simulink model "topic_sub"  (R2020b)
settings: Solver=FixedStepAuto  StartTime=0.0  StopTime=inf  RelTol=1e-3
undefined symbols (not defined in the file): BodyRate, Header, Orientation, Pose, Twist
libraries: robotlib x33, pid_lib x4
settings Model: Creator=mario  LastModifiedBy=mario
settings OptimizationCC: DefaultParameterBehavior=Inlined  EnhancedBackFolding=on  PassReuseOutputArgsAs=Individual arguments  ZeroExternalMemoryAtStartup=off  ZeroInternalMemoryAtStartup=off  InitFltsAndDblsToZero=on  MaxStackSize=64  OptimizeBlockOrder=speed  DifferentSizesBufferReuse=on  OptimizationCustomize=off  EfficientTunableParamExpr=on
settings DebuggingCC: ParameterTunabilityLossMsg=error
settings HardwareCC: ProdBitPerPointer=32  ProdBitPerSizeT=32  ProdBitPerPtrDiffT=32  ProdLargestAtomicFloat=None  ProdIntDivRoundTo=Undefined  ProdEndianess=Unspecified  ProdWordSize=32  ProdLongLongMode=on  ProdHWDeviceType=Generic->Unspecified (assume 32-bit Generic)  TargetLongLongMode=on
settings SFSimCC: MATLABDynamicMemAlloc=off
settings RTWCC: Description=Embedded Coder  SystemTargetFile=ert.tlc  HardwareBoard=Robot Operating System (ROS)  TLCOptions="-aInlineSetEventsForThisBaseRateFcn=TLC_FALSE -aSuppressMultiTaskScheduler=TLC_FALSE  -aRateBasedStepFcn=0"  GenCodeOnly=on  TemplateMakefile=ert_default_tmf  Toolchain=Catkin  TargetLang=C++  GenerateGPUCode=CUDA
settings CodeAppCC: ForceParamTrailComments=on  IgnoreCustomStorageClasses=off  OperatorAnnotations=on  SimulinkDataObjDesc=on  SFDataObjDesc=on  InsertBlockDesc=on
settings ERTTargetCC: CodeInterfacePackaging=C++ class  InlinedParameterPlacement=NonHierarchical  RootIOFormat=Structure reference  ERTCustomFileTemplate=example_file_process.tlc

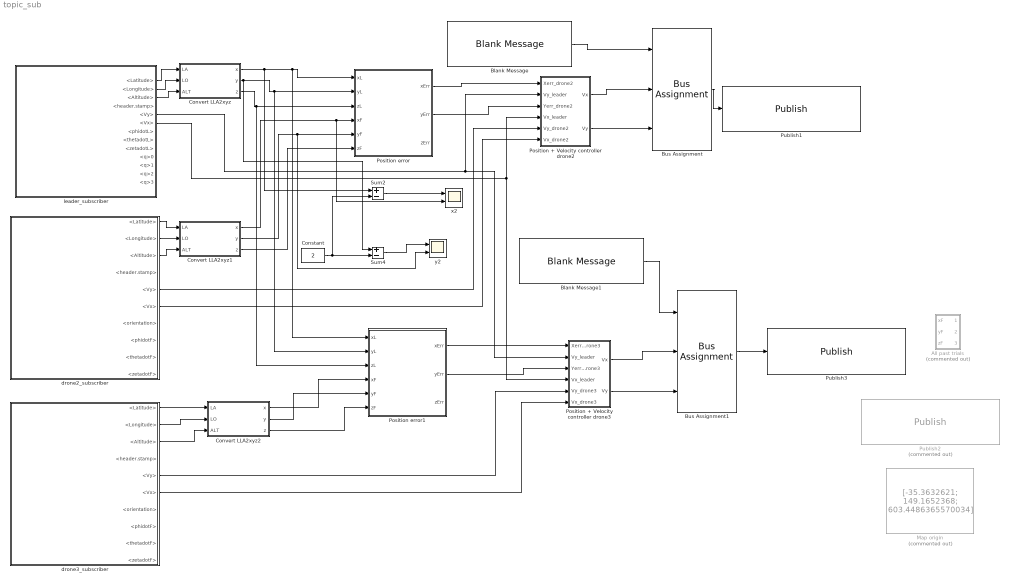
== system topic_sub ==
  All past trials : Subsystem  Commented=on
  Blank Message : robotlib/Blank Message  messageClass=Message  entityType=geometry_msgs/TwistStamped  messageType=geometry_msgs/TwistStamped  SampleTime=inf  legacyBusStruct=off
  Blank Message1 : robotlib/Blank Message  messageClass=Message  entityType=geometry_msgs/TwistStamped  messageType=geometry_msgs/TwistStamped  SampleTime=inf  legacyBusStruct=off
  Bus Assignment : BusAssignment  AssignedSignals=Twist.Linear.X,Twist.Linear.Y
  Bus Assignment1 : BusAssignment  AssignedSignals=Twist.Linear.X,Twist.Linear.Y
  Constant : Constant  Value=2
  Convert LLA2xyz : MATLAB Function  TreatAsAtomicUnit=on
  Convert LLA2xyz1 : MATLAB Function  TreatAsAtomicUnit=on
  Convert LLA2xyz2 : MATLAB Function  TreatAsAtomicUnit=on
  Map origin : Constant  Commented=on  Value=[-35.3632621; 149.1652368; 603.4486365570034]  VectorParams1D=off  SampleTime=-1
  Position + Velocity controller drone2 : Subsystem
  Position + Velocity controller drone3 : Subsystem
  Position error : MATLAB Function  TreatAsAtomicUnit=on
  Position error1 : MATLAB Function  TreatAsAtomicUnit=on
  Publish1 : robotlib/Publish  topicSource=Select from ROS network  topic=/drone2/mavros/setpoint_velocity/cmd_vel  messageType=geometry_msgs/TwistStamped  legacyBusStruct=off  messageQueueLength=1
  Publish2 : robotlib/Publish  Commented=on  topicSource=Select from ROS network  topic=/drone2/mavros/setpoint_velocity/cmd_vel  messageType=geometry_msgs/TwistStamped  legacyBusStruct=off  messageQueueLength=1
  Publish3 : robotlib/Publish  topicSource=Select from ROS network  topic=/drone3/mavros/setpoint_velocity/cmd_vel  messageType=geometry_msgs/TwistStamped  legacyBusStruct=off  messageQueueLength=1
  Sum2 : Sum  Inputs=+-
  Sum4 : Sum  Inputs=+-
  drone2_subscriber : Subsystem
  drone3_subscriber : Subsystem
  leader_subscriber : Subsystem
  x2 : Scope  NumInputPorts=2
  y2 : Scope  NumInputPorts=2
  wires:
  Blank Message/1 -> Bus Assignment/1
  Bus Assignment/1 -> Publish1/1
  leader_subscriber/1(<Latitude>) -> Convert LLA2xyz/1(LA)
  leader_subscriber/2(<Longitude>) -> Convert LLA2xyz/2(LO)
  leader_subscriber/3(<Altitude>) -> Convert LLA2xyz/3(ALT)
  Convert LLA2xyz/1(x) -> Sum2/1, Position error1/1(xL), Position error/1(xL)
  Convert LLA2xyz/2(y) -> Sum4/1, Position error1/2(yL), Position error/2(yL)
  Convert LLA2xyz/3(z) -> Position error1/3(zL), Position error/3(zL)
  drone2_subscriber/2(<Longitude>) -> Convert LLA2xyz1/2(LO)
  drone2_subscriber/1(<Latitude>) -> Convert LLA2xyz1/1(LA)
  drone2_subscriber/3(<Altitude>) -> Convert LLA2xyz1/3(ALT)
  Convert LLA2xyz1/1(x) -> x2/2, Position error/4(xF)
  Convert LLA2xyz1/2(y) -> Position error/5(yF), y2/2
  Convert LLA2xyz1/3(z) -> Position error/6(zF)
  Constant/1 -> Sum2/2, Sum4/2
  Position error/1(xErr) -> Position + Velocity controller drone2/1(Xerr_drone2)
  leader_subscriber/5(<Vy>) -> Position + Velocity controller drone2/2(Vy_leader), Position + Velocity controller drone3/2(Vy_leader)
  Position error/2(yErr) -> Position + Velocity controller drone2/3(Yerr_drone2)
  leader_subscriber/6(<Vx>) -> Position + Velocity controller drone3/4(Vx_leader), Position + Velocity controller drone2/4(Vx_leader)
  drone2_subscriber/5(<Vy>) -> Position + Velocity controller drone2/5(Vy_drone2)
  drone2_subscriber/6(<Vx>) -> Position + Velocity controller drone2/6(Vx_drone2)
  Position + Velocity controller drone2/1(Vx) -> Bus Assignment/2
  Position + Velocity controller drone2/2(Vy) -> Bus Assignment/3
  Sum2/1 -> x2/1
  Sum4/1 -> y2/1
  drone3_subscriber/1(<Latitude>) -> Convert LLA2xyz2/1(LA)
  drone3_subscriber/2(<Longitude>) -> Convert LLA2xyz2/2(LO)
  drone3_subscriber/3(<Altitude>) -> Convert LLA2xyz2/3(ALT)
  Convert LLA2xyz2/1(x) -> Position error1/4(xF)
  Convert LLA2xyz2/2(y) -> Position error1/5(yF)
  Convert LLA2xyz2/3(z) -> Position error1/6(zF)
  Position error1/1(xErr) -> Position + Velocity controller drone3/1(Xerr_drone3)
  Position error1/2(yErr) -> Position + Velocity controller drone3/3(Yerr_drone3)
  Position + Velocity controller drone3/1(Vx) -> Bus Assignment1/2
  Position + Velocity controller drone3/2(Vy) -> Bus Assignment1/3
  Bus Assignment1/1 -> Publish3/1
  Blank Message1/1 -> Bus Assignment1/1
  drone3_subscriber/5(<Vy>) -> Position + Velocity controller drone3/5(Vy_drone3)
  drone3_subscriber/6(<Vx>) -> Position + Velocity controller drone3/6(Vx_drone3)

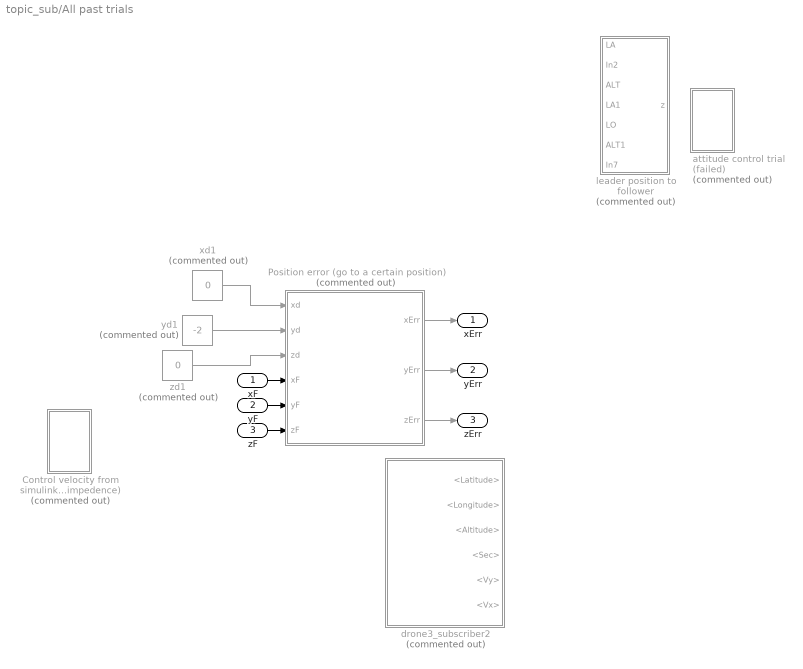
== system topic_sub/All past trials ==
  xF : Inport
  yF : Inport  Port=2
  zF : Inport  Port=3
  Control velocity from simulink trial(virtual impedence) : Subsystem  Commented=on
  Position error (go to a certain position) : MATLAB Function  Commented=on  TreatAsAtomicUnit=on
  attitude control trial (failed) : Subsystem  Commented=on
  drone3_subscriber2 : Subsystem  Commented=on
  leader position to follower : Subsystem  Commented=on
  xd1 : Constant  Commented=on  Value=0
  yd1 : Constant  Commented=on  Value=-2
  zd1 : Constant  Commented=on  Value=0
  xErr : Outport
  yErr : Outport  Port=2
  zErr : Outport  Port=3
  wires:
  Position error (go to a certain position)/3(zErr) -> zErr/1
  Position error (go to a certain position)/2(yErr) -> yErr/1
  xF/1 -> Position error (go to a certain position)/4(xF)
  zF/1 -> Position error (go to a certain position)/6(zF)
  yd1/1 -> Position error (go to a certain position)/2(yd)
  xd1/1 -> Position error (go to a certain position)/1(xd)
  Position error (go to a certain position)/1(xErr) -> xErr/1
  yF/1 -> Position error (go to a certain position)/5(yF)
  zd1/1 -> Position error (go to a certain position)/3(zd)

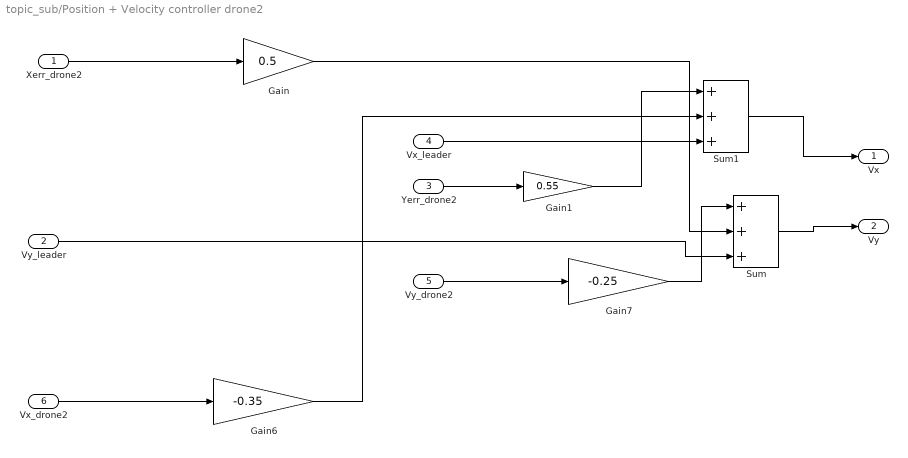
== system topic_sub/Position + Velocity controller drone2 ==
  Xerr_drone2 : Inport
  Vy_leader : Inport  Port=2
  Yerr_drone2 : Inport  Port=3
  Vx_leader : Inport  Port=4
  Vy_drone2 : Inport  Port=5
  Vx_drone2 : Inport  Port=6
  Gain : Gain  Gain=0.5
  Gain1 : Gain  Gain=0.55
  Gain6 : Gain  Gain=-0.35
  Gain7 : Gain  Gain=-0.25
  Sum : Sum  Inputs=+++
  Sum1 : Sum  Inputs=+++
  Vx : Outport
  Vy : Outport  Port=2
  wires:
  Vx_leader/1 -> Sum1/3
  Vy_leader/1 -> Sum/3
  Gain6/1 -> Sum1/2
  Vy_drone2/1 -> Gain7/1
  Gain7/1 -> Sum/1
  Sum/1 -> Vy/1
  Sum1/1 -> Vx/1
  Xerr_drone2/1 -> Gain/1
  Yerr_drone2/1 -> Gain1/1
  Gain1/1 -> Sum1/1
  Vx_drone2/1 -> Gain6/1
  Gain/1 -> Sum/2

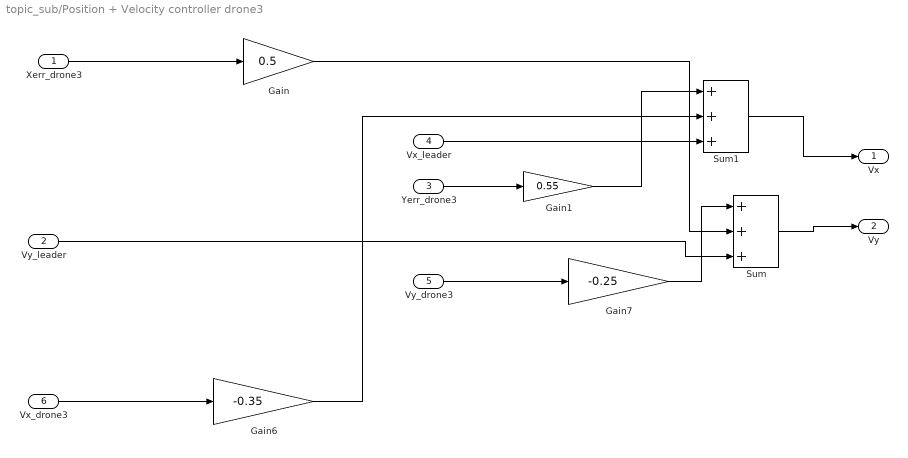
== system topic_sub/Position + Velocity controller drone3 ==
  Xerr_drone3 : Inport
  Vy_leader : Inport  Port=2
  Yerr_drone3 : Inport  Port=3
  Vx_leader : Inport  Port=4
  Vy_drone3 : Inport  Port=5
  Vx_drone3 : Inport  Port=6
  Gain : Gain  Gain=0.5
  Gain1 : Gain  Gain=0.55
  Gain6 : Gain  Gain=-0.35
  Gain7 : Gain  Gain=-0.25
  Sum : Sum  Inputs=+++
  Sum1 : Sum  Inputs=+++
  Vx : Outport
  Vy : Outport  Port=2
  wires:
  Gain/1 -> Sum/2
  Vx_drone3/1 -> Gain6/1
  Gain1/1 -> Sum1/1
  Yerr_drone3/1 -> Gain1/1
  Xerr_drone3/1 -> Gain/1
  Sum1/1 -> Vx/1
  Sum/1 -> Vy/1
  Gain7/1 -> Sum/1
  Vy_drone3/1 -> Gain7/1
  Gain6/1 -> Sum1/2
  Vy_leader/1 -> Sum/3
  Vx_leader/1 -> Sum1/3

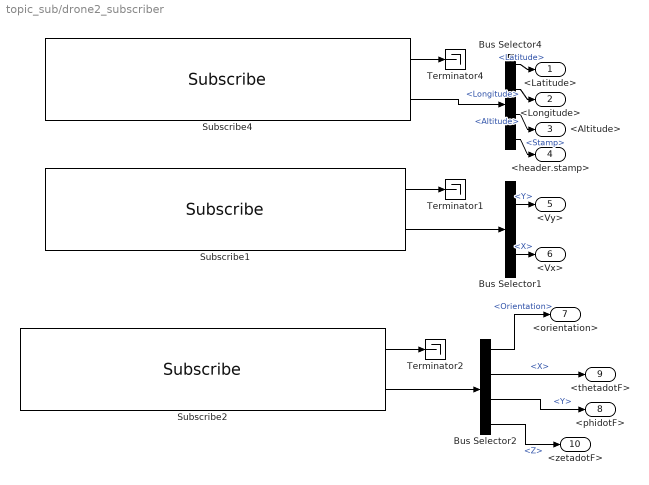
== system topic_sub/drone2_subscriber ==
  Bus Selector1 : BusSelector  OutputSignals=Twist.Linear.Y,Twist.Linear.X
  Bus Selector2 : BusSelector  OutputSignals=Orientation,AngularVelocity.X,AngularVelocity.Y,AngularVelocity.Z
  Bus Selector4 : BusSelector  OutputSignals=Latitude,Longitude,Altitude,Header.Stamp
  Subscribe1 : robotlib/Subscribe  topicSource=Select from ROS network  topic=/drone2/mavros/global_position/raw/gps_vel  messageType=geometry_msgs/TwistStamped  SampleTime=-1  legacyBusStruct=off  messageQueueLength=1
  Subscribe2 : robotlib/Subscribe  topicSource=Select from ROS network  topic=/drone2/mavros/imu/data  messageType=sensor_msgs/Imu  SampleTime=-1  legacyBusStruct=off  messageQueueLength=1
  Subscribe4 : robotlib/Subscribe  topicSource=Select from ROS network  topic=/drone2/mavros/global_position/raw/fix  messageType=sensor_msgs/NavSatFix  SampleTime=-1  legacyBusStruct=off  messageQueueLength=1
  Terminator1 : Terminator
  Terminator2 : Terminator
  Terminator4 : Terminator
  <Latitude> : Outport
  <Longitude> : Outport  Port=2
  <Altitude> : Outport  Port=3
  <header.stamp> : Outport  Port=4
  <Vy> : Outport  Port=5
  <Vx> : Outport  Port=6
  <orientation> : Outport  Port=7
  <phidotF> : Outport  Port=8
  <thetadotF> : Outport  Port=9
  <zetadotF> : Outport  Port=10
  wires:
  Bus Selector4/1 -> <Latitude>/1  "<Latitude>"
  Subscribe1/2 -> Bus Selector1/1
  Bus Selector1/2 -> <Vx>/1  "<X>"
  Subscribe4/1 -> Terminator4/1
  Bus Selector1/1 -> <Vy>/1  "<Y>"
  Bus Selector4/3 -> <Altitude>/1  "<Altitude>"
  Bus Selector4/2 -> <Longitude>/1  "<Longitude>"
  Subscribe1/1 -> Terminator1/1
  Subscribe4/2 -> Bus Selector4/1
  Bus Selector2/3 -> <phidotF>/1  "<Y>"
  Bus Selector2/4 -> <zetadotF>/1  "<Z>"
  Subscribe2/2 -> Bus Selector2/1
  Subscribe2/1 -> Terminator2/1
  Bus Selector2/2 -> <thetadotF>/1  "<X>"
  Bus Selector2/1 -> <orientation>/1  "<Orientation>"
  Bus Selector4/4 -> <header.stamp>/1  "<Stamp>"

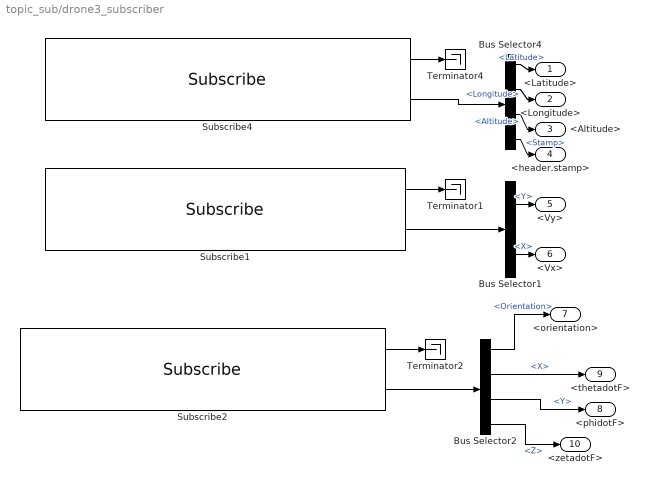
== system topic_sub/drone3_subscriber ==
  Bus Selector1 : BusSelector  OutputSignals=Twist.Linear.Y,Twist.Linear.X
  Bus Selector2 : BusSelector  OutputSignals=Orientation,AngularVelocity.X,AngularVelocity.Y,AngularVelocity.Z
  Bus Selector4 : BusSelector  OutputSignals=Latitude,Longitude,Altitude,Header.Stamp
  Subscribe1 : robotlib/Subscribe  topicSource=Select from ROS network  topic=/drone3/mavros/global_position/raw/gps_vel  messageType=geometry_msgs/TwistStamped  SampleTime=-1  legacyBusStruct=off  messageQueueLength=1
  Subscribe2 : robotlib/Subscribe  topicSource=Select from ROS network  topic=/drone3/mavros/imu/data  messageType=sensor_msgs/Imu  SampleTime=-1  legacyBusStruct=off  messageQueueLength=1
  Subscribe4 : robotlib/Subscribe  topicSource=Select from ROS network  topic=/drone3/mavros/global_position/raw/fix  messageType=sensor_msgs/NavSatFix  SampleTime=-1  legacyBusStruct=off  messageQueueLength=1
  Terminator1 : Terminator
  Terminator2 : Terminator
  Terminator4 : Terminator
  <Latitude> : Outport
  <Longitude> : Outport  Port=2
  <Altitude> : Outport  Port=3
  <header.stamp> : Outport  Port=4
  <Vy> : Outport  Port=5
  <Vx> : Outport  Port=6
  <orientation> : Outport  Port=7
  <phidotF> : Outport  Port=8
  <thetadotF> : Outport  Port=9
  <zetadotF> : Outport  Port=10
  wires:
  Bus Selector4/4 -> <header.stamp>/1  "<Stamp>"
  Bus Selector2/1 -> <orientation>/1  "<Orientation>"
  Bus Selector2/2 -> <thetadotF>/1  "<X>"
  Subscribe2/1 -> Terminator2/1
  Subscribe2/2 -> Bus Selector2/1
  Bus Selector2/4 -> <zetadotF>/1  "<Z>"
  Bus Selector2/3 -> <phidotF>/1  "<Y>"
  Subscribe4/2 -> Bus Selector4/1
  Subscribe1/1 -> Terminator1/1
  Bus Selector4/2 -> <Longitude>/1  "<Longitude>"
  Bus Selector4/3 -> <Altitude>/1  "<Altitude>"
  Bus Selector1/1 -> <Vy>/1  "<Y>"
  Subscribe4/1 -> Terminator4/1
  Bus Selector1/2 -> <Vx>/1  "<X>"
  Subscribe1/2 -> Bus Selector1/1
  Bus Selector4/1 -> <Latitude>/1  "<Latitude>"

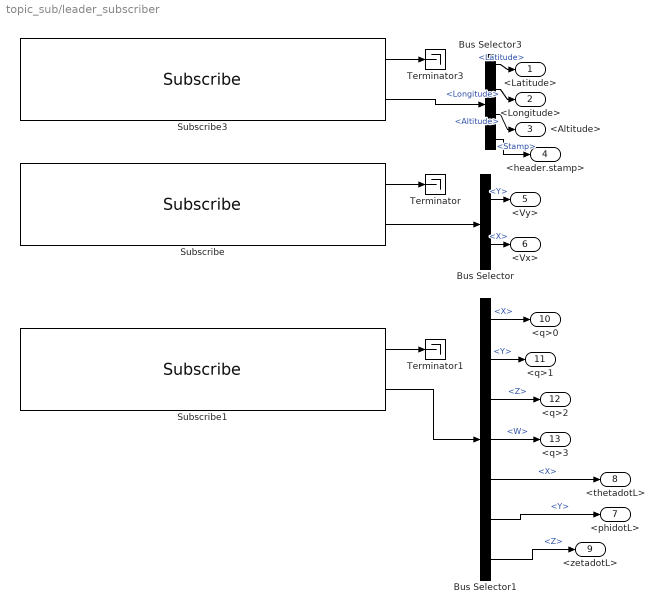
== system topic_sub/leader_subscriber ==
  Bus Selector : BusSelector  OutputSignals=Twist.Linear.Y,Twist.Linear.X
  Bus Selector1 : BusSelector  OutputSignals=Orientation.X,Orientation.Y,Orientation.Z,Orientation.W,AngularVelocity.X,AngularVelocity.Y,AngularVelocity.Z
  Bus Selector3 : BusSelector  OutputSignals=Latitude,Longitude,Altitude,Header.Stamp
  Subscribe : robotlib/Subscribe  topicSource=Select from ROS network  topic=/drone1/mavros/global_position/raw/gps_vel  messageType=geometry_msgs/TwistStamped  SampleTime=-1  legacyBusStruct=off  messageQueueLength=1
  Subscribe1 : robotlib/Subscribe  topicSource=Select from ROS network  topic=/drone1/mavros/imu/data  messageType=sensor_msgs/Imu  SampleTime=-1  legacyBusStruct=off  messageQueueLength=1
  Subscribe3 : robotlib/Subscribe  topicSource=Select from ROS network  topic=/drone1/mavros/global_position/raw/fix  messageType=sensor_msgs/NavSatFix  SampleTime=-1  legacyBusStruct=off  messageQueueLength=1000
  Terminator : Terminator
  Terminator1 : Terminator
  Terminator3 : Terminator
  <Latitude> : Outport
  <Longitude> : Outport  Port=2
  <Altitude> : Outport  Port=3
  <header.stamp> : Outport  Port=4
  <Vy> : Outport  Port=5
  <Vx> : Outport  Port=6
  <phidotL> : Outport  Port=7
  <thetadotL> : Outport  Port=8
  <zetadotL> : Outport  Port=9
  <q>0 : Outport  Port=10
  <q>1 : Outport  Port=11
  <q>2 : Outport  Port=12
  <q>3 : Outport  Port=13
  wires:
  Bus Selector3/3 -> <Altitude>/1  "<Altitude>"
  Subscribe3/1 -> Terminator3/1
  Subscribe3/2 -> Bus Selector3/1
  Bus Selector3/2 -> <Longitude>/1  "<Longitude>"
  Bus Selector/2 -> <Vx>/1  "<X>"
  Bus Selector3/1 -> <Latitude>/1  "<Latitude>"
  Subscribe/2 -> Bus Selector/1
  Bus Selector/1 -> <Vy>/1  "<Y>"
  Subscribe/1 -> Terminator/1
  Subscribe1/1 -> Terminator1/1
  Subscribe1/2 -> Bus Selector1/1
  Bus Selector1/5 -> <thetadotL>/1  "<X>"
  Bus Selector1/6 -> <phidotL>/1  "<Y>"
  Bus Selector1/7 -> <zetadotL>/1  "<Z>"
  Bus Selector1/1 -> <q>0/1  "<X>"
  Bus Selector1/2 -> <q>1/1  "<Y>"
  Bus Selector1/3 -> <q>2/1  "<Z>"
  Bus Selector1/4 -> <q>3/1  "<W>"
  Bus Selector3/4 -> <header.stamp>/1  "<Stamp>"

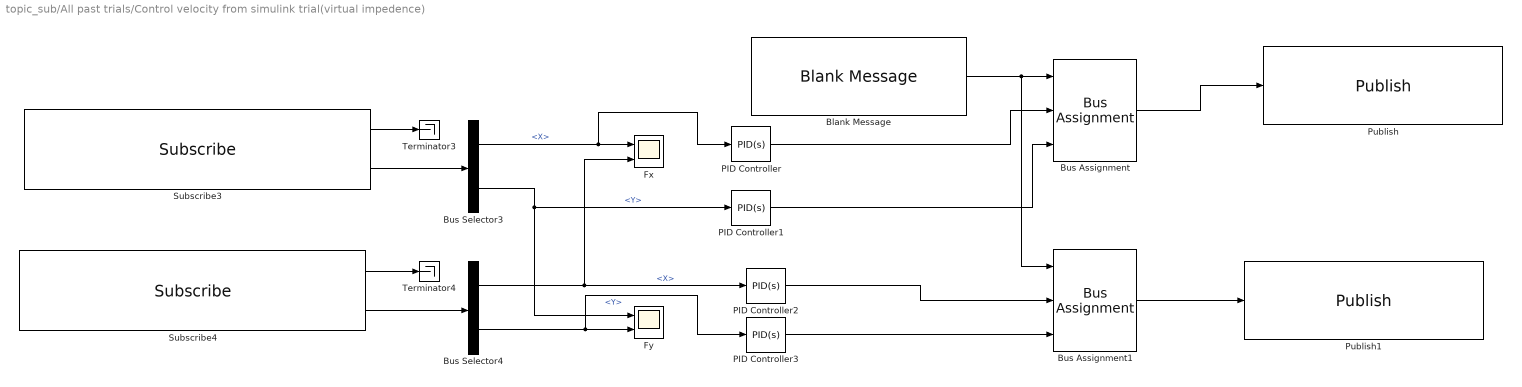
== system topic_sub/All past trials/Control velocity from simulink trial(virtual impedence) ==
  Blank Message : robotlib/Blank Message  messageClass=Message  entityType=geometry_msgs/TwistStamped  messageType=geometry_msgs/TwistStamped  SampleTime=inf  legacyBusStruct=off
  Bus Assignment : BusAssignment  AssignedSignals=Twist.Linear.X,Twist.Linear.Y
  Bus Assignment1 : BusAssignment  AssignedSignals=Twist.Linear.X,Twist.Linear.Y
  Bus Selector3 : BusSelector  OutputSignals=Vector.X,Vector.Y
  Bus Selector4 : BusSelector  OutputSignals=Vector.X,Vector.Y
  Fx : Scope  NumInputPorts=2
  Fy : Scope  NumInputPorts=2
  PID Controller : pid_lib/PID Controller  Controller=PID  Form=Parallel  TimeDomain=Continuous-time  UseExternalTs=off  SampleTime=-1  IntegratorMethod=Forward Euler  FilterMethod=Forward Euler  ControllerParametersSource=internal  P=1  I=1  D=1  UseFilter=on  N=1  TunerSelectOption=Frequency Response Based  InitialConditionSource=internal  InitialConditionForIntegrator=0  InitialConditionForFilter=0  DifferentiatorICPrevScaledInput=0  ExternalReset=none  TrackingMode=off  Kt=1  LimitOutput=off  SatLimitsSource=internal  UpperSaturationLimit=inf  LowerSaturationLimit=-inf  LinearizeAsGain=on  AntiWindupMode=none  Kb=1  POutMin=[]  POutMax=[]  IOutMin=[]  IOutMax=[]  DOutMin=[]  DOutMax=[]  NOutMin=[]  NOutMax=[]  SumOutMin=[]  SumOutMax=[]  SaturationOutMin=[]  SaturationOutMax=[]  PParamMin=[]  PParamMax=[]  IParamMin=[]  IParamMax=[]  DParamMin=[]  DParamMax=[]  NParamMin=[]  NParamMax=[]  KbParamMin=[]  KbParamMax=[]  KtParamMin=[]  KtParamMax=[]  KbOutMin=[]  KbOutMax=[]  KtOutMin=[]  KtOutMax=[]  IntegratorOutMin=[]  IntegratorOutMax=[]  FilterOutMin=[]  FilterOutMax=[]  SumI1OutMin=[]  SumI1OutMax=[]  SumI2OutMin=[]  SumI2OutMax=[]  SumI3OutMin=[]  SumI3OutMax=[]  SumI4OutMin=[]  SumI4OutMax=[]  SumDOutMin=[]  SumDOutMax=[]  DifferentiatorOutMin=[]  DifferentiatorOutMax=[]  FilterDiffOutCoefMin=[]  FilterDiffOutCoefMax=[]  ReciprocalOutMin=[]  ReciprocalOutMax=[]  SumDenOutMin=[]  SumDenOutMax=[]  SumNumOutMin=[]  SumNumOutMax=[]  DivideOutMin=[]  DivideOutMax=[]  UdiffTsProdOutMin=[]  UdiffTsProdOutMax=[]  NTsProdOutMin=[]  NTsProdOutMax=[]  UintegralTsProdOutMin=[]  UintegralTsProdOutMax=[]  UngainTsProdOutMin=[]  UngainTsProdOutMax=[]  IntegratorContinuousStateAttributes=''  IntegratorStateMustResolveToSignalObject=off  IntegratorRTWStateStorageClass=Auto  FilterContinuousStateAttributes=''  FilterStateMustResolveToSignalObject=off  FilterRTWStateStorageClass=Auto  ParallelPVariant=InternalParameters  IdealPVariant=Disabled  IVariant=InternalParameters  DVariant=InternalParameters  IntegratorVariant=Continuous  SatVariant=Disabled  AWVariant=Passthrough  PCopyVariant=Disabled  TRVariant=Disabled  FdbkBlocksVariant=Forward  IdealPFdbkVariant=Disabled  SatFdbkVariant=Disabled  DerivativeFilterVariant=ContFilter  NVariant=InternalParameters  NCopyVariant=Disabled  FilterICVariant=InternalICsFilter  IntegratorICVariant=InternalICs  ExternalResetVariant=Disabled  TRSumVariant=Passthrough  SumFdbkVariant=Disabled  SumVariant=Sum_PID  TsampFilterVariant=InternalTs  TsampNgainVariant=Passthrough  TsampIntegralVariant=Passthrough  ExternalSaturationOutDataTypeStr=Inherit: Same as second input
  PID Controller1 : pid_lib/PID Controller  Controller=PID  Form=Parallel  TimeDomain=Continuous-time  UseExternalTs=off  SampleTime=-1  IntegratorMethod=Forward Euler  FilterMethod=Forward Euler  ControllerParametersSource=internal  P=1  I=1  D=0  UseFilter=on  N=100  TunerSelectOption=Transfer Function Based (PID Tuner App)  InitialConditionSource=internal  InitialConditionForIntegrator=0  InitialConditionForFilter=0  DifferentiatorICPrevScaledInput=0  ExternalReset=none  TrackingMode=off  Kt=1  LimitOutput=off  SatLimitsSource=internal  UpperSaturationLimit=inf  LowerSaturationLimit=-inf  LinearizeAsGain=on  AntiWindupMode=none  Kb=1  POutMin=[]  POutMax=[]  IOutMin=[]  IOutMax=[]  DOutMin=[]  DOutMax=[]  NOutMin=[]  NOutMax=[]  SumOutMin=[]  SumOutMax=[]  SaturationOutMin=[]  SaturationOutMax=[]  PParamMin=[]  PParamMax=[]  IParamMin=[]  IParamMax=[]  DParamMin=[]  DParamMax=[]  NParamMin=[]  NParamMax=[]  KbParamMin=[]  KbParamMax=[]  KtParamMin=[]  KtParamMax=[]  KbOutMin=[]  KbOutMax=[]  KtOutMin=[]  KtOutMax=[]  IntegratorOutMin=[]  IntegratorOutMax=[]  FilterOutMin=[]  FilterOutMax=[]  SumI1OutMin=[]  SumI1OutMax=[]  SumI2OutMin=[]  SumI2OutMax=[]  SumI3OutMin=[]  SumI3OutMax=[]  SumI4OutMin=[]  SumI4OutMax=[]  SumDOutMin=[]  SumDOutMax=[]  DifferentiatorOutMin=[]  DifferentiatorOutMax=[]  FilterDiffOutCoefMin=[]  FilterDiffOutCoefMax=[]  ReciprocalOutMin=[]  ReciprocalOutMax=[]  SumDenOutMin=[]  SumDenOutMax=[]  SumNumOutMin=[]  SumNumOutMax=[]  DivideOutMin=[]  DivideOutMax=[]  UdiffTsProdOutMin=[]  UdiffTsProdOutMax=[]  NTsProdOutMin=[]  NTsProdOutMax=[]  UintegralTsProdOutMin=[]  UintegralTsProdOutMax=[]  UngainTsProdOutMin=[]  UngainTsProdOutMax=[]  IntegratorContinuousStateAttributes=''  IntegratorStateMustResolveToSignalObject=off  IntegratorRTWStateStorageClass=Auto  FilterContinuousStateAttributes=''  FilterStateMustResolveToSignalObject=off  FilterRTWStateStorageClass=Auto  ParallelPVariant=InternalParameters  IdealPVariant=Disabled  IVariant=InternalParameters  DVariant=InternalParameters  IntegratorVariant=Continuous  SatVariant=Disabled  AWVariant=Passthrough  PCopyVariant=Disabled  TRVariant=Disabled  FdbkBlocksVariant=Forward  IdealPFdbkVariant=Disabled  SatFdbkVariant=Disabled  DerivativeFilterVariant=ContFilter  NVariant=InternalParameters  NCopyVariant=Disabled  FilterICVariant=InternalICsFilter  IntegratorICVariant=InternalICs  ExternalResetVariant=Disabled  TRSumVariant=Passthrough  SumFdbkVariant=Disabled  SumVariant=Sum_PID  TsampFilterVariant=InternalTs  TsampNgainVariant=Passthrough  TsampIntegralVariant=Passthrough  ExternalSaturationOutDataTypeStr=Inherit: Same as second input
  PID Controller2 : pid_lib/PID Controller  Controller=PID  Form=Parallel  TimeDomain=Continuous-time  UseExternalTs=off  SampleTime=-1  IntegratorMethod=Forward Euler  FilterMethod=Forward Euler  ControllerParametersSource=internal  P=1  I=1  D=0  UseFilter=on  N=100  TunerSelectOption=Transfer Function Based (PID Tuner App)  InitialConditionSource=internal  InitialConditionForIntegrator=0  InitialConditionForFilter=0  DifferentiatorICPrevScaledInput=0  ExternalReset=none  TrackingMode=off  Kt=1  LimitOutput=off  SatLimitsSource=internal  UpperSaturationLimit=inf  LowerSaturationLimit=-inf  LinearizeAsGain=on  AntiWindupMode=none  Kb=1  POutMin=[]  POutMax=[]  IOutMin=[]  IOutMax=[]  DOutMin=[]  DOutMax=[]  NOutMin=[]  NOutMax=[]  SumOutMin=[]  SumOutMax=[]  SaturationOutMin=[]  SaturationOutMax=[]  PParamMin=[]  PParamMax=[]  IParamMin=[]  IParamMax=[]  DParamMin=[]  DParamMax=[]  NParamMin=[]  NParamMax=[]  KbParamMin=[]  KbParamMax=[]  KtParamMin=[]  KtParamMax=[]  KbOutMin=[]  KbOutMax=[]  KtOutMin=[]  KtOutMax=[]  IntegratorOutMin=[]  IntegratorOutMax=[]  FilterOutMin=[]  FilterOutMax=[]  SumI1OutMin=[]  SumI1OutMax=[]  SumI2OutMin=[]  SumI2OutMax=[]  SumI3OutMin=[]  SumI3OutMax=[]  SumI4OutMin=[]  SumI4OutMax=[]  SumDOutMin=[]  SumDOutMax=[]  DifferentiatorOutMin=[]  DifferentiatorOutMax=[]  FilterDiffOutCoefMin=[]  FilterDiffOutCoefMax=[]  ReciprocalOutMin=[]  ReciprocalOutMax=[]  SumDenOutMin=[]  SumDenOutMax=[]  SumNumOutMin=[]  SumNumOutMax=[]  DivideOutMin=[]  DivideOutMax=[]  UdiffTsProdOutMin=[]  UdiffTsProdOutMax=[]  NTsProdOutMin=[]  NTsProdOutMax=[]  UintegralTsProdOutMin=[]  UintegralTsProdOutMax=[]  UngainTsProdOutMin=[]  UngainTsProdOutMax=[]  IntegratorContinuousStateAttributes=''  IntegratorStateMustResolveToSignalObject=off  IntegratorRTWStateStorageClass=Auto  FilterContinuousStateAttributes=''  FilterStateMustResolveToSignalObject=off  FilterRTWStateStorageClass=Auto  ParallelPVariant=InternalParameters  IdealPVariant=Disabled  IVariant=InternalParameters  DVariant=InternalParameters  IntegratorVariant=Continuous  SatVariant=Disabled  AWVariant=Passthrough  PCopyVariant=Disabled  TRVariant=Disabled  FdbkBlocksVariant=Forward  IdealPFdbkVariant=Disabled  SatFdbkVariant=Disabled  DerivativeFilterVariant=ContFilter  NVariant=InternalParameters  NCopyVariant=Disabled  FilterICVariant=InternalICsFilter  IntegratorICVariant=InternalICs  ExternalResetVariant=Disabled  TRSumVariant=Passthrough  SumFdbkVariant=Disabled  SumVariant=Sum_PID  TsampFilterVariant=InternalTs  TsampNgainVariant=Passthrough  TsampIntegralVariant=Passthrough  ExternalSaturationOutDataTypeStr=Inherit: Same as second input
  PID Controller3 : pid_lib/PID Controller  Controller=PID  Form=Parallel  TimeDomain=Continuous-time  UseExternalTs=off  SampleTime=-1  IntegratorMethod=Forward Euler  FilterMethod=Forward Euler  ControllerParametersSource=internal  P=1  I=1  D=0  UseFilter=on  N=100  TunerSelectOption=Transfer Function Based (PID Tuner App)  InitialConditionSource=internal  InitialConditionForIntegrator=0  InitialConditionForFilter=0  DifferentiatorICPrevScaledInput=0  ExternalReset=none  TrackingMode=off  Kt=1  LimitOutput=off  SatLimitsSource=internal  UpperSaturationLimit=inf  LowerSaturationLimit=-inf  LinearizeAsGain=on  AntiWindupMode=none  Kb=1  POutMin=[]  POutMax=[]  IOutMin=[]  IOutMax=[]  DOutMin=[]  DOutMax=[]  NOutMin=[]  NOutMax=[]  SumOutMin=[]  SumOutMax=[]  SaturationOutMin=[]  SaturationOutMax=[]  PParamMin=[]  PParamMax=[]  IParamMin=[]  IParamMax=[]  DParamMin=[]  DParamMax=[]  NParamMin=[]  NParamMax=[]  KbParamMin=[]  KbParamMax=[]  KtParamMin=[]  KtParamMax=[]  KbOutMin=[]  KbOutMax=[]  KtOutMin=[]  KtOutMax=[]  IntegratorOutMin=[]  IntegratorOutMax=[]  FilterOutMin=[]  FilterOutMax=[]  SumI1OutMin=[]  SumI1OutMax=[]  SumI2OutMin=[]  SumI2OutMax=[]  SumI3OutMin=[]  SumI3OutMax=[]  SumI4OutMin=[]  SumI4OutMax=[]  SumDOutMin=[]  SumDOutMax=[]  DifferentiatorOutMin=[]  DifferentiatorOutMax=[]  FilterDiffOutCoefMin=[]  FilterDiffOutCoefMax=[]  ReciprocalOutMin=[]  ReciprocalOutMax=[]  SumDenOutMin=[]  SumDenOutMax=[]  SumNumOutMin=[]  SumNumOutMax=[]  DivideOutMin=[]  DivideOutMax=[]  UdiffTsProdOutMin=[]  UdiffTsProdOutMax=[]  NTsProdOutMin=[]  NTsProdOutMax=[]  UintegralTsProdOutMin=[]  UintegralTsProdOutMax=[]  UngainTsProdOutMin=[]  UngainTsProdOutMax=[]  IntegratorContinuousStateAttributes=''  IntegratorStateMustResolveToSignalObject=off  IntegratorRTWStateStorageClass=Auto  FilterContinuousStateAttributes=''  FilterStateMustResolveToSignalObject=off  FilterRTWStateStorageClass=Auto  ParallelPVariant=InternalParameters  IdealPVariant=Disabled  IVariant=InternalParameters  DVariant=InternalParameters  IntegratorVariant=Continuous  SatVariant=Disabled  AWVariant=Passthrough  PCopyVariant=Disabled  TRVariant=Disabled  FdbkBlocksVariant=Forward  IdealPFdbkVariant=Disabled  SatFdbkVariant=Disabled  DerivativeFilterVariant=ContFilter  NVariant=InternalParameters  NCopyVariant=Disabled  FilterICVariant=InternalICsFilter  IntegratorICVariant=InternalICs  ExternalResetVariant=Disabled  TRSumVariant=Passthrough  SumFdbkVariant=Disabled  SumVariant=Sum_PID  TsampFilterVariant=InternalTs  TsampNgainVariant=Passthrough  TsampIntegralVariant=Passthrough  ExternalSaturationOutDataTypeStr=Inherit: Same as second input
  Publish : robotlib/Publish  topicSource=Select from ROS network  topic=/drone2/mavros/setpoint_velocity/cmd_vel  messageType=geometry_msgs/TwistStamped  legacyBusStruct=off  messageQueueLength=1
  Publish1 : robotlib/Publish  topicSource=Select from ROS network  topic=/drone3/mavros/setpoint_velocity/cmd_vel  messageType=geometry_msgs/TwistStamped  legacyBusStruct=off  messageQueueLength=1
  Subscribe3 : robotlib/Subscribe  topicSource=Select from ROS network  topic=/drone2/impedence_force  messageType=geometry_msgs/Vector3Stamped  SampleTime=-1  legacyBusStruct=off  messageQueueLength=1
  Subscribe4 : robotlib/Subscribe  topicSource=Select from ROS network  topic=/drone3/impedence_force  messageType=geometry_msgs/Vector3Stamped  SampleTime=-1  legacyBusStruct=off  messageQueueLength=1
  Terminator3 : Terminator
  Terminator4 : Terminator
  wires:
  PID Controller/1 -> Bus Assignment/2
  Bus Assignment1/1 -> Publish1/1
  Bus Selector4/2 -> PID Controller3/1, Fy/2  "<Y>"
  Bus Selector4/1 -> Fx/2, PID Controller2/1  "<X>"
  Subscribe4/2 -> Bus Selector4/1
  Bus Selector3/1 -> PID Controller/1, Fx/1  "<X>"
  Bus Selector3/2 -> Fy/1, PID Controller1/1  "<Y>"
  Subscribe3/2 -> Bus Selector3/1
  Subscribe3/1 -> Terminator3/1
  Blank Message/1 -> Bus Assignment1/1, Bus Assignment/1
  Subscribe4/1 -> Terminator4/1
  PID Controller3/1 -> Bus Assignment1/3
  PID Controller1/1 -> Bus Assignment/3
  Bus Assignment/1 -> Publish/1
  PID Controller2/1 -> Bus Assignment1/2

== system topic_sub/All past trials/attitude control trial (failed) ==
  formation control failed trial : Subsystem  Commented=on
  set attitude : Subsystem  Commented=on

== system topic_sub/All past trials/drone3_subscriber2 ==
  Bus Selector2 : BusSelector  OutputSignals=Header.Stamp.Sec,Twist.Linear.Y,Twist.Linear.X
  Bus Selector5 : BusSelector  OutputSignals=Latitude,Longitude,Altitude
  Subscribe2 : robotlib/Subscribe  topicSource=Select from ROS network  topic=/drone3/mavros/global_position/raw/gps_vel  messageType=geometry_msgs/TwistStamped  SampleTime=-1  legacyBusStruct=off  messageQueueLength=1
  Subscribe5 : robotlib/Subscribe  topicSource=Select from ROS network  topic=/drone3/mavros/global_position/raw/fix  messageType=sensor_msgs/NavSatFix  SampleTime=-1  legacyBusStruct=off  messageQueueLength=1
  Terminator2 : Terminator
  Terminator5 : Terminator
  <Latitude> : Outport
  <Longitude> : Outport  Port=2
  <Altitude> : Outport  Port=3
  <Sec> : Outport  Port=4
  <Vy> : Outport  Port=5
  <Vx> : Outport  Port=6
  wires:
  Bus Selector2/1 -> <Sec>/1  "<Sec>"
  Bus Selector2/3 -> <Vx>/1  "<X>"
  Bus Selector2/2 -> <Vy>/1  "<Y>"
  Bus Selector5/1 -> <Latitude>/1  "<Latitude>"
  Subscribe5/2 -> Bus Selector5/1
  Bus Selector5/2 -> <Longitude>/1  "<Longitude>"
  Subscribe2/1 -> Terminator2/1
  Bus Selector5/3 -> <Altitude>/1  "<Altitude>"
  Subscribe2/2 -> Bus Selector2/1
  Subscribe5/1 -> Terminator5/1

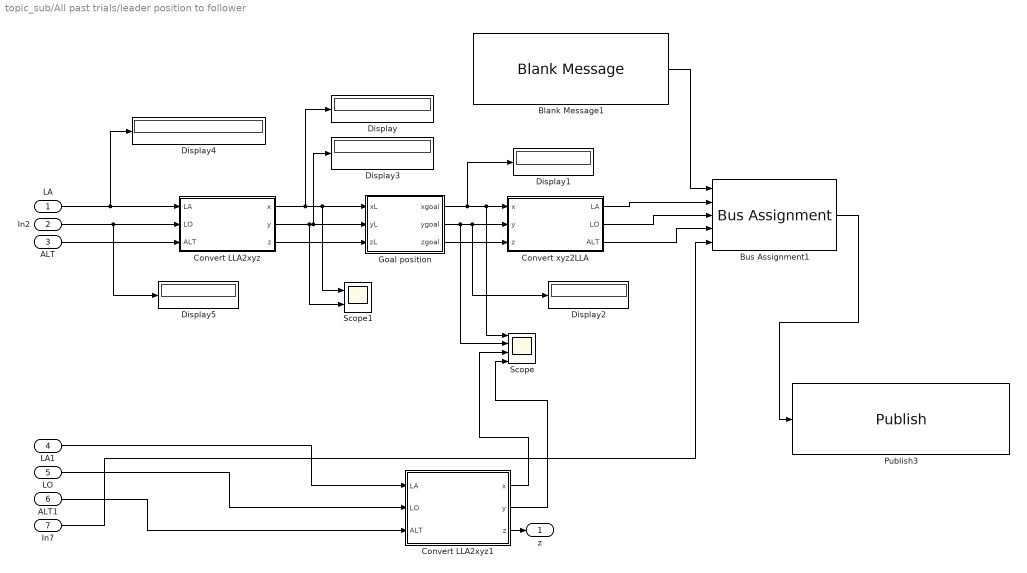
== system topic_sub/All past trials/leader position to follower ==
  LA : Inport
  In2 : Inport  Port=2
  ALT : Inport  Port=3
  LA1 : Inport  Port=4
  LO : Inport  Port=5
  ALT1 : Inport  Port=6
  In7 : Inport  Port=7
  Blank Message1 : robotlib/Blank Message  messageClass=Message  entityType=geographic_msgs/GeoPoseStamped  messageType=geographic_msgs/GeoPoseStamped  SampleTime=inf  legacyBusStruct=off
  Bus Assignment1 : BusAssignment  AssignedSignals=Pose.Position.Latitude,Pose.Position.Longitude,Pose.Position.Altitude,Header.Stamp
  Convert LLA2xyz : MATLAB Function  TreatAsAtomicUnit=on
  Convert LLA2xyz1 : MATLAB Function  TreatAsAtomicUnit=on
  Convert xyz2LLA : MATLAB Function  TreatAsAtomicUnit=on
  Display{,1..5} (6 alike) : Display
      Display4 settings: Decimation=5
  Goal position : MATLAB Function  TreatAsAtomicUnit=on
  Publish3 : robotlib/Publish  topicSource=Select from ROS network  topic=/drone2/mavros/setpoint_position/global  messageType=geographic_msgs/GeoPoseStamped  legacyBusStruct=off  messageQueueLength=1000
  Scope : Scope  NumInputPorts=4
  Scope1 : Scope  NumInputPorts=2
  z : Outport
  wires:
  In7/1 -> Bus Assignment1/5
  Bus Assignment1/1 -> Publish3/1
  Convert xyz2LLA/1(LA) -> Bus Assignment1/2
  Blank Message1/1 -> Bus Assignment1/1
  Convert LLA2xyz1/1(x) -> Scope/3
  ALT1/1 -> Convert LLA2xyz1/3(ALT)
  Convert xyz2LLA/3(ALT) -> Bus Assignment1/4
  LA/1 -> Convert LLA2xyz/1(LA), Display4/1
  In2/1 -> Display5/1, Convert LLA2xyz/2(LO)
  ALT/1 -> Convert LLA2xyz/3(ALT)
  Convert LLA2xyz/2(y) -> Scope1/2, Goal position/2(yL), Display3/1
  Convert LLA2xyz1/3(z) -> z/1
  Goal position/1(xgoal) -> Display1/1, Scope/1, Convert xyz2LLA/1(x)
  Convert LLA2xyz1/2(y) -> Scope/4
  Convert LLA2xyz/3(z) -> Goal position/3(zL)
  Goal position/2(ygoal) -> Scope/2, Display2/1, Convert xyz2LLA/2(y)
  LO/1 -> Convert LLA2xyz1/2(LO)
  LA1/1 -> Convert LLA2xyz1/1(LA)
  Convert xyz2LLA/2(LO) -> Bus Assignment1/3
  Convert LLA2xyz/1(x) -> Display/1, Scope1/1, Goal position/1(xL)
  Goal position/3(zgoal) -> Convert xyz2LLA/3(z)

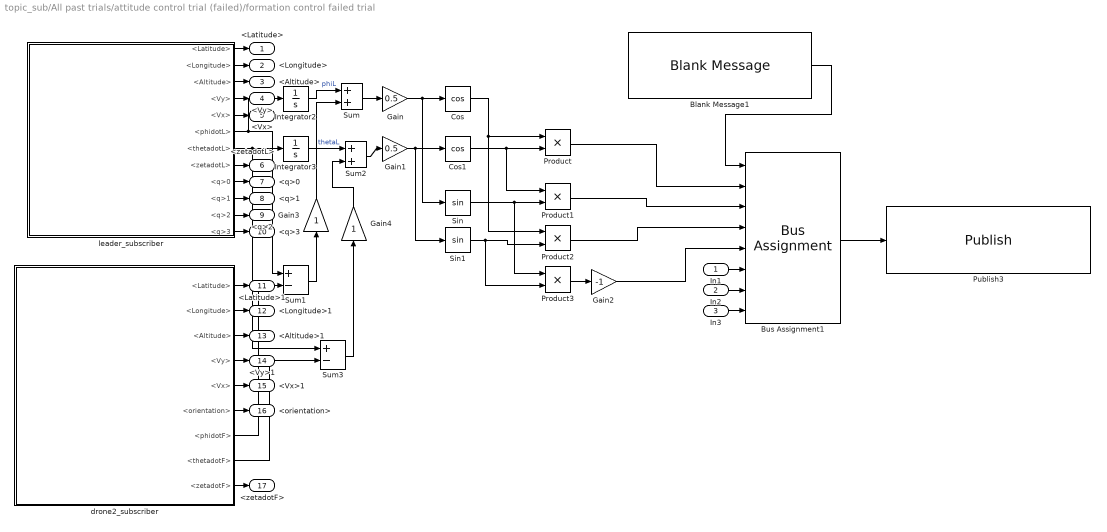
== system topic_sub/All past trials/attitude control trial (failed)/formation control failed trial ==
  In1 : Inport
  In2 : Inport  Port=2
  In3 : Inport  Port=3
  Blank Message1 : robotlib/Blank Message  messageClass=Message  entityType=mavros_msgs/AttitudeTarget  messageType=mavros_msgs/AttitudeTarget  SampleTime=inf  legacyBusStruct=off
  Bus Assignment1 : BusAssignment  AssignedSignals=Orientation.X,Orientation.Y,Orientation.Z,Orientation.W,BodyRate.X,BodyRate.Y,BodyRate.Z
  Cos : Trigonometry  Operator=cos
  Cos1 : Trigonometry  Operator=cos
  Gain : Gain  Gain=0.5
  Gain1 : Gain  Gain=0.5
  Gain2 : Gain  Gain=-1
  Gain3 : Gain
  Gain4 : Gain
  Integrator2 : Integrator
  Integrator3 : Integrator
  Product{,1..3} (4 alike) : Product
  Publish3 : robotlib/Publish  topicSource=Select from ROS network  topic=/drone2/mavros/setpoint_raw/attitude  messageType=mavros_msgs/AttitudeTarget  legacyBusStruct=off  messageQueueLength=1
  Sin : Trigonometry
  Sin1 : Trigonometry
  Sum : Sum
  Sum1 : Sum  Inputs=+-
  Sum2 : Sum
  Sum3 : Sum  Inputs=+-
  drone2_subscriber : Subsystem
  leader_subscriber : Subsystem
  <Latitude> : Outport
  <Longitude> : Outport  Port=2
  <Altitude> : Outport  Port=3
  <Vy> : Outport  Port=4
  <Vx> : Outport  Port=5
  <zetadotL> : Outport  Port=6
  <q>0 : Outport  Port=7
  <q>1 : Outport  Port=8
  <q>2 : Outport  Port=9
  <q>3 : Outport  Port=10
  <Latitude>1 : Outport  Port=11
  <Longitude>1 : Outport  Port=12
  <Altitude>1 : Outport  Port=13
  <Vy>1 : Outport  Port=14
  <Vx>1 : Outport  Port=15
  <orientation> : Outport  Port=16
  <zetadotF> : Outport  Port=17
  wires:
  In1/1 -> Bus Assignment1/6
  drone2_subscriber/1(<Latitude>) -> <Latitude>1/1
  drone2_subscriber/5(<Vx>) -> <Vx>1/1
  leader_subscriber/12(<q>3) -> <q>3/1
  leader_subscriber/5(<Vx>) -> <Vx>/1
  drone2_subscriber/4(<Vy>) -> <Vy>1/1
  Sum1/1 -> Gain3/1
  Product/1 -> Bus Assignment1/2
  Product3/1 -> Gain2/1
  leader_subscriber/7(<thetadotL>) -> Sum3/1, Integrator3/1
  Sum/1 -> Gain/1
  Bus Assignment1/1 -> Publish3/1
  leader_subscriber/9(<q>0) -> <q>0/1
  leader_subscriber/8(<zetadotL>) -> <zetadotL>/1
  Sum3/1 -> Gain4/1
  Product1/1 -> Bus Assignment1/3
  Sum2/1 -> Gain1/1
  Gain1/1 -> Sin1/1, Cos1/1
  Integrator3/1 -> Sum2/1  "thetaL"
  Gain4/1 -> Sum2/2
  Sin/1 -> Product3/1, Product1/2
  Sin1/1 -> Product3/2, Product2/2
  leader_subscriber/3(<Altitude>) -> <Altitude>/1
  Gain/1 -> Sin/1, Cos/1
  Gain2/1 -> Bus Assignment1/5
  Cos/1 -> Product2/1, Product/1
  Gain3/1 -> Sum/2
  drone2_subscriber/2(<Longitude>) -> <Longitude>1/1
  In3/1 -> Bus Assignment1/8
  drone2_subscriber/7(<phidotF>) -> Sum1/2
  Product2/1 -> Bus Assignment1/4
  drone2_subscriber/3(<Altitude>) -> <Altitude>1/1
  Integrator2/1 -> Sum/1  "phiL"
  drone2_subscriber/9(<zetadotF>) -> <zetadotF>/1
  drone2_subscriber/6(<orientation>) -> <orientation>/1
  drone2_subscriber/8(<thetadotF>) -> Sum3/2
  In2/1 -> Bus Assignment1/7
  Blank Message1/1 -> Bus Assignment1/1
  Cos1/1 -> Product1/1, Product/2
  leader_subscriber/2(<Longitude>) -> <Longitude>/1
  leader_subscriber/10(<q>1) -> <q>1/1
  leader_subscriber/1(<Latitude>) -> <Latitude>/1
  leader_subscriber/6(<phidotL>) -> Sum1/1, Integrator2/1
  leader_subscriber/4(<Vy>) -> <Vy>/1
  leader_subscriber/11(<q>2) -> <q>2/1

== system topic_sub/All past trials/attitude control trial (failed)/set attitude ==
  In1 : Inport
  In2 : Inport  Port=2
  In3 : Inport  Port=3
  In4 : Inport  Port=4
  In5 : Inport  Port=5
  In6 : Inport  Port=6
  In7 : Inport  Port=7
  Blank Message1 : robotlib/Blank Message  messageClass=Message  entityType=mavros_msgs/AttitudeTarget  messageType=mavros_msgs/AttitudeTarget  SampleTime=inf  legacyBusStruct=off
  Bus Assignment1 : BusAssignment  AssignedSignals=Orientation.X,Orientation.Y,Orientation.Z,Orientation.W,BodyRate.X,BodyRate.Y,BodyRate.Z
  Publish3 : robotlib/Publish  topicSource=Select from ROS network  topic=/drone2/mavros/setpoint_raw/attitude  messageType=mavros_msgs/AttitudeTarget  legacyBusStruct=off  messageQueueLength=1
  wires:
  In1/1 -> Bus Assignment1/6
  In5/1 -> Bus Assignment1/3
  Bus Assignment1/1 -> Publish3/1
  Blank Message1/1 -> Bus Assignment1/1
  In7/1 -> Bus Assignment1/5
  In4/1 -> Bus Assignment1/2
  In3/1 -> Bus Assignment1/8
  In2/1 -> Bus Assignment1/7
  In6/1 -> Bus Assignment1/4

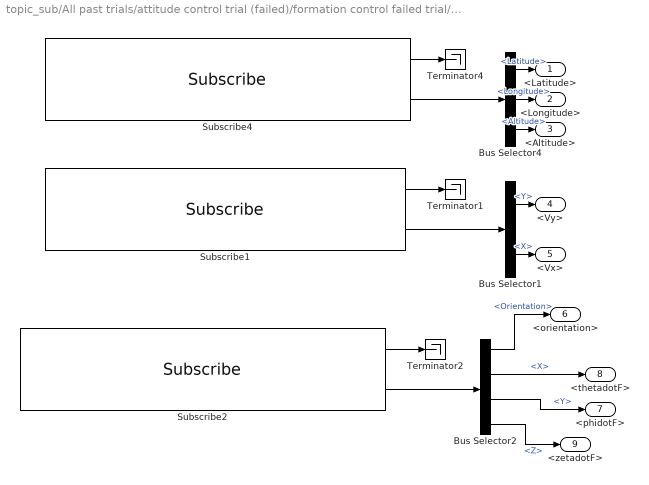
== system topic_sub/All past trials/attitude control trial (failed)/formation control failed trial/drone2_subscriber ==
  Bus Selector1 : BusSelector  OutputSignals=Twist.Linear.Y,Twist.Linear.X
  Bus Selector2 : BusSelector  OutputSignals=Orientation,AngularVelocity.X,AngularVelocity.Y,AngularVelocity.Z
  Bus Selector4 : BusSelector  OutputSignals=Latitude,Longitude,Altitude
  Subscribe1 : robotlib/Subscribe  topicSource=Select from ROS network  topic=/drone2/mavros/global_position/raw/gps_vel  messageType=geometry_msgs/TwistStamped  SampleTime=-1  legacyBusStruct=off  messageQueueLength=1
  Subscribe2 : robotlib/Subscribe  topicSource=Select from ROS network  topic=/drone2/mavros/imu/data  messageType=sensor_msgs/Imu  SampleTime=-1  legacyBusStruct=off  messageQueueLength=1
  Subscribe4 : robotlib/Subscribe  topicSource=Select from ROS network  topic=/drone2/mavros/global_position/raw/fix  messageType=sensor_msgs/NavSatFix  SampleTime=-1  legacyBusStruct=off  messageQueueLength=1
  Terminator1 : Terminator
  Terminator2 : Terminator
  Terminator4 : Terminator
  <Latitude> : Outport
  <Longitude> : Outport  Port=2
  <Altitude> : Outport  Port=3
  <Vy> : Outport  Port=4
  <Vx> : Outport  Port=5
  <orientation> : Outport  Port=6
  <phidotF> : Outport  Port=7
  <thetadotF> : Outport  Port=8
  <zetadotF> : Outport  Port=9
  wires:
  Bus Selector4/1 -> <Latitude>/1  "<Latitude>"
  Subscribe1/2 -> Bus Selector1/1
  Bus Selector1/2 -> <Vx>/1  "<X>"
  Subscribe4/1 -> Terminator4/1
  Bus Selector1/1 -> <Vy>/1  "<Y>"
  Bus Selector4/3 -> <Altitude>/1  "<Altitude>"
  Bus Selector4/2 -> <Longitude>/1  "<Longitude>"
  Subscribe1/1 -> Terminator1/1
  Subscribe4/2 -> Bus Selector4/1
  Bus Selector2/3 -> <phidotF>/1  "<Y>"
  Bus Selector2/4 -> <zetadotF>/1  "<Z>"
  Subscribe2/2 -> Bus Selector2/1
  Subscribe2/1 -> Terminator2/1
  Bus Selector2/2 -> <thetadotF>/1  "<X>"
  Bus Selector2/1 -> <orientation>/1  "<Orientation>"

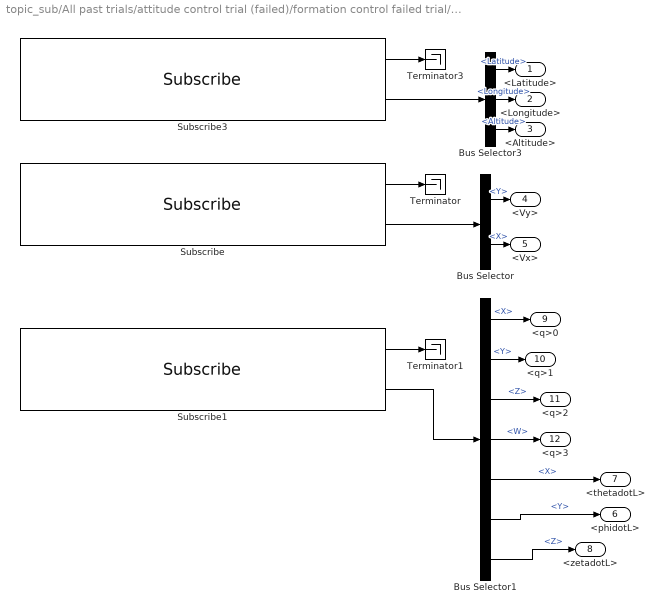
== system topic_sub/All past trials/attitude control trial (failed)/formation control failed trial/leader_subscriber ==
  Bus Selector : BusSelector  OutputSignals=Twist.Linear.Y,Twist.Linear.X
  Bus Selector1 : BusSelector  OutputSignals=Orientation.X,Orientation.Y,Orientation.Z,Orientation.W,AngularVelocity.X,AngularVelocity.Y,AngularVelocity.Z
  Bus Selector3 : BusSelector  OutputSignals=Latitude,Longitude,Altitude
  Subscribe : robotlib/Subscribe  topicSource=Select from ROS network  topic=/drone1/mavros/global_position/raw/gps_vel  messageType=geometry_msgs/TwistStamped  SampleTime=-1  legacyBusStruct=off  messageQueueLength=1
  Subscribe1 : robotlib/Subscribe  topicSource=Select from ROS network  topic=/drone1/mavros/imu/data  messageType=sensor_msgs/Imu  SampleTime=-1  legacyBusStruct=off  messageQueueLength=1
  Subscribe3 : robotlib/Subscribe  topicSource=Select from ROS network  topic=/drone1/mavros/global_position/raw/fix  messageType=sensor_msgs/NavSatFix  SampleTime=-1  legacyBusStruct=off  messageQueueLength=1
  Terminator : Terminator
  Terminator1 : Terminator
  Terminator3 : Terminator
  <Latitude> : Outport
  <Longitude> : Outport  Port=2
  <Altitude> : Outport  Port=3
  <Vy> : Outport  Port=4
  <Vx> : Outport  Port=5
  <phidotL> : Outport  Port=6
  <thetadotL> : Outport  Port=7
  <zetadotL> : Outport  Port=8
  <q>0 : Outport  Port=9
  <q>1 : Outport  Port=10
  <q>2 : Outport  Port=11
  <q>3 : Outport  Port=12
  wires:
  Bus Selector3/3 -> <Altitude>/1  "<Altitude>"
  Subscribe3/1 -> Terminator3/1
  Subscribe3/2 -> Bus Selector3/1
  Bus Selector3/2 -> <Longitude>/1  "<Longitude>"
  Bus Selector/2 -> <Vx>/1  "<X>"
  Bus Selector3/1 -> <Latitude>/1  "<Latitude>"
  Subscribe/2 -> Bus Selector/1
  Bus Selector/1 -> <Vy>/1  "<Y>"
  Subscribe/1 -> Terminator/1
  Subscribe1/1 -> Terminator1/1
  Subscribe1/2 -> Bus Selector1/1
  Bus Selector1/5 -> <thetadotL>/1  "<X>"
  Bus Selector1/6 -> <phidotL>/1  "<Y>"
  Bus Selector1/7 -> <zetadotL>/1  "<Z>"
  Bus Selector1/1 -> <q>0/1  "<X>"
  Bus Selector1/2 -> <q>1/1  "<Y>"
  Bus Selector1/3 -> <q>2/1  "<Z>"
  Bus Selector1/4 -> <q>3/1  "<W>"

== matlab function topic_sub/Convert LLA2xyz2 ==
  data: LA input; x output; LO input; ALT input; y output; z output
function [x,y,z]= fcn(LA , LO, ALT)

x = (LA -(-35.3632621)) * 10^5 ;
y = (LO -(149.1652368)) * 10^5 ;
z = ALT- (603.4486365570034);

== matlab function topic_sub/All past trials/Position error (go to a certain position) ==
  data: xd input; xErr output; yd input; zd input; yErr output; zErr output; xF input; yF input; zF input
function [xErr , yErr, zErr]= fcn(xd,yd,zd,xF,yF,zF)

xErr = xd - xF ;
yErr = yd - yF ;
zErr = zd - zF;

== matlab function topic_sub/All past trials/leader position to follower/Convert xyz2LLA ==
  data: x input; LA output; y input; z input; LO output; ALT output
function [LA , LO, ALT]= fcn(x,y,z)

LA  = (x  * 10^-5) + (-35.3632621);
LO  = (y  * 10^-5) + (149.1652368);
ALT = z  + (603.4486365570034) - 19.5;

== matlab function topic_sub/All past trials/leader position to follower/Convert LLA2xyz ==
  data: LA input; x output; LO input; ALT input; y output; z output
function [x,y,z]= fcn(LA , LO, ALT)

x = (LA -(-35.3632621)) * 10^5 ;
y = (LO -(149.1652368)) * 10^5 ;
z = ALT- (603.4486365570034);

== matlab function topic_sub/All past trials/leader position to follower/Goal position ==
  data: xL input; xgoal output; yL input; zL input; ygoal output; zgoal output
function [xgoal , ygoal, zgoal]= fcn(xL,yL,zL)

xgoal = xL - 2;
ygoal = yL - 2;
zgoal = zL;

== matlab function topic_sub/Position error ==
  data: xL input; xErr output; yL input; zL input; yErr output; zErr output; xF input; yF input; zF input
function [xErr , yErr, zErr]= fcn(xL,yL,zL,xF,yF,zF)
xd = 2;
yd = 2;
xErr = xL - xF - xd;
yErr = yL - yF - yd;
zErr = zL - zF;

== matlab function topic_sub/All past trials/leader position to follower/Convert LLA2xyz1 ==
  data: LA input; x output; LO input; ALT input; y output; z output
function [x,y,z]= fcn(LA , LO, ALT)

x = (LA -(-35.3632621)) * 10^5 ;
y = (LO -(149.1652368)) * 10^5 ;
z = ALT- (603.4486365570034);

== matlab function topic_sub/Convert LLA2xyz ==
  data: LA input; x output; LO input; ALT input; y output; z output
function [x,y,z]= fcn(LA , LO, ALT)

x = (LA -(-35.3632621)) * 10^5 ;
y = (LO -(149.1652368)) * 10^5 ;
z = ALT- (603.4486365570034);

== matlab function topic_sub/Position error1 ==
  data: xL input; xErr output; yL input; zL input; yErr output; zErr output; xF input; yF input; zF input
function [xErr , yErr, zErr]= fcn(xL,yL,zL,xF,yF,zF)
xd = 2;
yd = -2;
xErr = xL - xF - xd;
yErr = yL - yF - yd;
zErr = zL - zF;

== matlab function topic_sub/Convert LLA2xyz1 ==
  data: LA input; x output; LO input; ALT input; y output; z output
function [x,y,z]= fcn(LA , LO, ALT)

x = (LA -(-35.3632621)) * 10^5 ;
y = (LO -(149.1652368)) * 10^5 ;
z = ALT- (603.4486365570034);
